simulink model "Nelinearni_system"  (R2020a)
settings: Solver=VariableStepAuto  StartTime=0.0  StopTime=10.0  RelTol=1e-3
values from neighbouring files (symbols this model uses):
  dphi = 0    [Model_kyvadla_na_voziku_m.m]
  dx = 0    [Model_kyvadla_na_voziku_m.m]
  f = 10    [Model_kyvadla_na_voziku_m.m]
  g = 9.81    [Model_kyvadla_na_voziku_m.m]
  l = 1    [Model_kyvadla_na_voziku_m.m]
  m = 5    [Model_kyvadla_na_voziku_m.m]
  M = 15    [Model_kyvadla_na_voziku_m.m]
  phi = deg2rad(1)    [Model_kyvadla_na_voziku_m.m]
  x = 0    [Model_kyvadla_na_voziku_m.m]
settings Model: Creator=Jiří  LastModifiedBy=Jiří

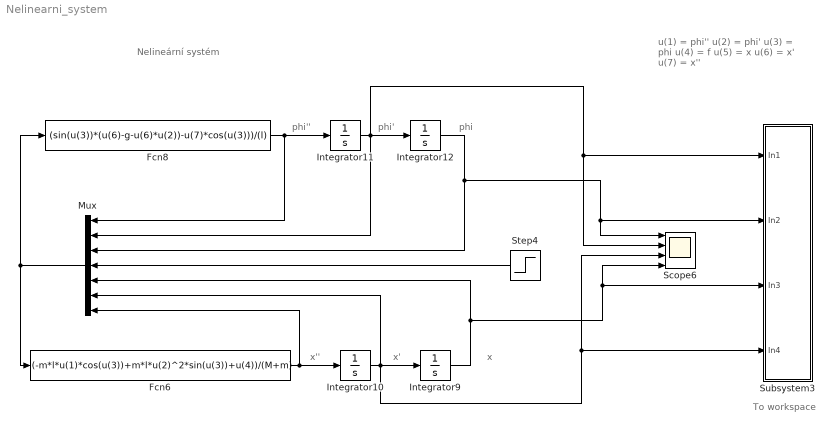
== system Nelinearni_system ==
  note: x''
  note: phi'
  note: x'
  note: x
  note: u(1) = phi''
      | u(2) = phi'
      | u(3) = phi
      | u(4) = f
      | u(5) = x
      | u(6) = x'
      | u(7) = x''
  note: phi''
  note: To workspace
  note: Nelineární systém
  note: phi
  Fcn6 : Fcn  Expr=(-m*l*u(1)*cos(u(3))+m*l*u(2)^2*sin(u(3))+u(4))/(M+m)
  Fcn8 : Fcn  Expr=(sin(u(3))*(u(6)-g-u(6)*u(2))-u(7)*cos(u(3)))/(l)
  Integrator10 : Integrator  InitialCondition=dx
  Integrator11 : Integrator  InitialCondition=dphi
  Integrator12 : Integrator  InitialCondition=phi
  Integrator9 : Integrator  InitialCondition=x
  Mux : Mux  Inputs=7
  Scope6 : Scope  NumInputPorts=4
  Step4 : Step  After=f  SampleTime=1
  Subsystem3 : Subsystem
  wires:
  Mux/1 -> Fcn8/1, Fcn6/1
  Step4/1 -> Mux/4
  Fcn8/1 -> Mux/1, Integrator11/1
  Integrator11/1 -> Integrator12/1, Scope6/2, Subsystem3/1(In1), Mux/2
  Fcn6/1 -> Mux/7, Integrator10/1
  Integrator10/1 -> Mux/6, Scope6/3, Subsystem3/4(In4), Integrator9/1
  Integrator9/1 -> Mux/5, Subsystem3/3(In3), Scope6/4
  Integrator12/1 -> Mux/3, Subsystem3/2(In2), Scope6/1

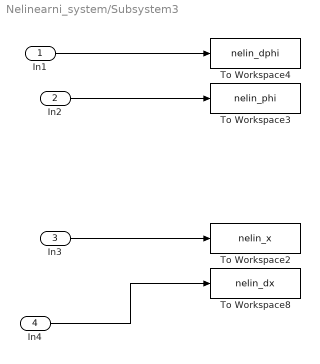
== system Nelinearni_system/Subsystem3 ==
  In1 : Inport
  In2 : Inport  Port=2
  In3 : Inport  Port=3
  In4 : Inport  Port=4
  To Workspace2 : ToWorkspace  VariableName=nelin_x  SaveFormat=Timeseries  SampleTime=-1
  To Workspace3 : ToWorkspace  VariableName=nelin_phi  SaveFormat=Timeseries  SampleTime=-1
  To Workspace4 : ToWorkspace  VariableName=nelin_dphi  SaveFormat=Timeseries  SampleTime=-1
  To Workspace8 : ToWorkspace  VariableName=nelin_dx  SaveFormat=Timeseries  SampleTime=-1
  wires:
  In4/1 -> To Workspace8/1
  In3/1 -> To Workspace2/1
  In2/1 -> To Workspace3/1
  In1/1 -> To Workspace4/1
